simulink model "ballbeampidsimulink2addingproposednonlinearitiesmodel"  (R2013b)
settings: Solver=ode45  StartTime=0.0  StopTime=500  RelTol=1e-3
values from neighbouring files (symbols this model uses):
  c = 3/5*9.8    (= 5.88)    [parametersofballsimuink.m]
  kd = 3/((180/pi)*(19.7/1.7))    (= 0.00451836506861)    [parametersofballsimuink.m]
  ki = 0.000/((180/pi)*(19.7/1.7))    (= 0)    [parametersofballsimuink.m]
  kp = 4/((180/pi)*(19.7/1.7))    (= 0.00602448675815)    [parametersofballsimuink.m]
  r = 20    [parametersofballsimuink.m]
settings Model: Creator=omar  LastModifiedBy=omar

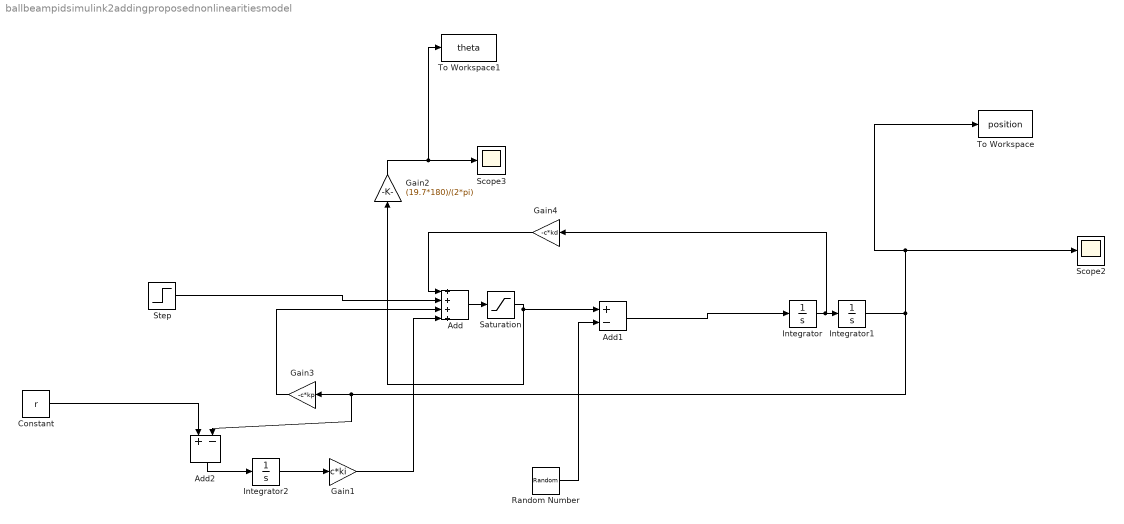
== system ballbeampidsimulink2addingproposednonlinearitiesmodel ==
  Add : Sum  Inputs=++++
  Add1 : Sum  Inputs=+-
  Add2 : Sum  Inputs=+-
  Constant : Constant  Value=r
  Gain1 : Gain  Gain=c*ki
  Gain2 : Gain  Gain=(19.7*180)/(2*pi)
  Gain3 : Gain  Gain=-c*kp
  Gain4 : Gain  Gain=-c*kd
  Integrator : Integrator
  Integrator1 : Integrator
  Integrator2 : Integrator
  Random Number : RandomNumber  Mean=0.03  Variance=0.01  SampleTime=0.1
  Saturation : Saturate  UpperLimit=0.124  LowerLimit=-0.124
  Scope2 : Scope
      settings: YMin=-30  YMax=10  SaveName=ScopeData2
  Scope3 : Scope
      settings: YMin=0  YMax=30  SaveName=ScopeData3
  Step : Step  Before=r*c*kp  After=r*c*kp  SampleTime=0
  To Workspace : ToWorkspace  VariableName=position  SampleTime=-1  SaveFormat=Timeseries
  To Workspace1 : ToWorkspace  VariableName=theta  SampleTime=-1  SaveFormat=Timeseries
  wires:
  Integrator/1 -> Gain4/1, Integrator1/1
  Integrator1/1 -> To Workspace/1, Scope2/1, Add2/2, Gain3/1
  Gain4/1 -> Add/1
  Gain3/1 -> Add/3
  Step/1 -> Add/2
  Gain2/1 -> To Workspace1/1, Scope3/1
  Add/1 -> Saturation/1
  Saturation/1 -> Add1/1, Gain2/1
  Random Number/1 -> Add1/2
  Add1/1 -> Integrator/1
  Add2/1 -> Integrator2/1
  Integrator2/1 -> Gain1/1
  Gain1/1 -> Add/4
  Constant/1 -> Add2/1
